simulink model "TST_TSDa_tClnt"  (R2016b)
settings: Solver=FixedStepDiscrete  StartTime=0.0  StopTime=simTime  FixedStep=sampleTime  RelTol=1e-3
values from neighbouring files (symbols this model uses):
  testCase = 1    [initTST_TSDa_tClnt_001.m]
libraries: simulink x5, UnitTest_Lib x3
settings Model: Creator=xinchangran  LastModifiedBy=xinchangran
settings DebuggingCC: SignalRangeChecking=error

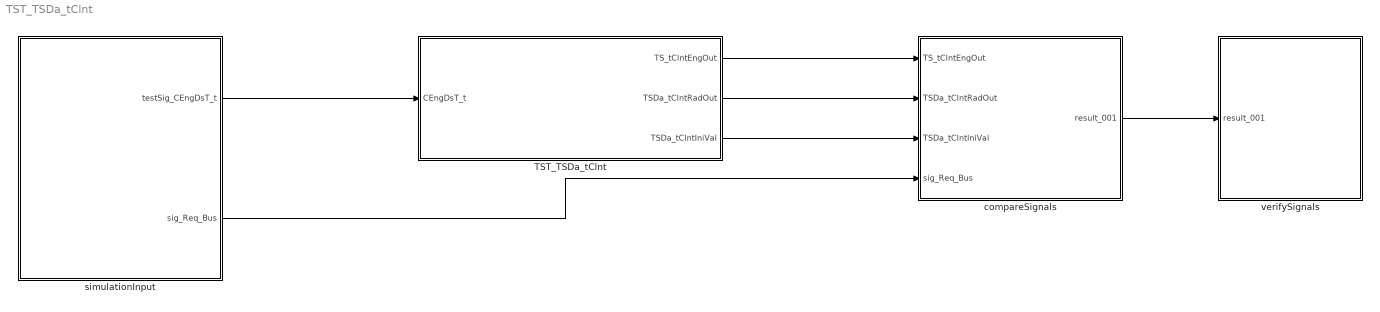
== system TST_TSDa_tClnt ==
  TST_TSDa_tClnt : Subsystem
  compareSignals : Subsystem
  simulationInput : Subsystem
  verifySignals : Subsystem
  wires:
  simulationInput/1(testSig_CEngDsT_t) -> TST_TSDa_tClnt/1(CEngDsT_t)
  TST_TSDa_tClnt/1(TS_tClntEngOut) -> compareSignals/1(TS_tClntEngOut)
  TST_TSDa_tClnt/2(TSDa_tClntRadOut) -> compareSignals/2(TSDa_tClntRadOut)
  TST_TSDa_tClnt/3(TSDa_tClntIniVal) -> compareSignals/3(TSDa_tClntIniVal)
  simulationInput/2(sig_Req_Bus) -> compareSignals/4(sig_Req_Bus)
  compareSignals/1(result_001) -> verifySignals/1(result_001)

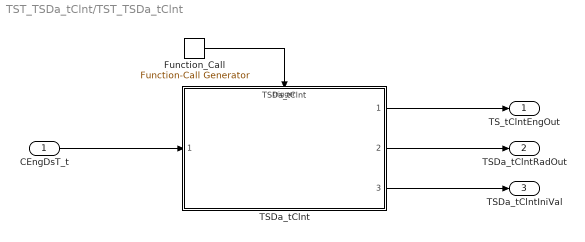
== system TST_TSDa_tClnt/TST_TSDa_tClnt ==
  CEngDsT_t : Inport
  Function_Call : simulink/Ports & Subsystems/Function-Call Generator  sample_time=sampleTime  numberOfIterations=1
  TSDa_tClnt : ModelReference  ModelNameDialog=TSDa_tClnt  SimulationMode=Normal  ModelReferenceVersion=1.10  TriggerPortName=function  TriggerPortTriggerType=function-call  TriggerPortStatesWhenEnabling=held
  TS_tClntEngOut : Outport
  TSDa_tClntRadOut : Outport  Port=2
  TSDa_tClntIniVal : Outport  Port=3
  wires:
  Function_Call/1 -> TSDa_tClnt/Trigger
  CEngDsT_t/1 -> TSDa_tClnt/1
  TSDa_tClnt/1 -> TS_tClntEngOut/1
  TSDa_tClnt/2 -> TSDa_tClntRadOut/1
  TSDa_tClnt/3 -> TSDa_tClntIniVal/1

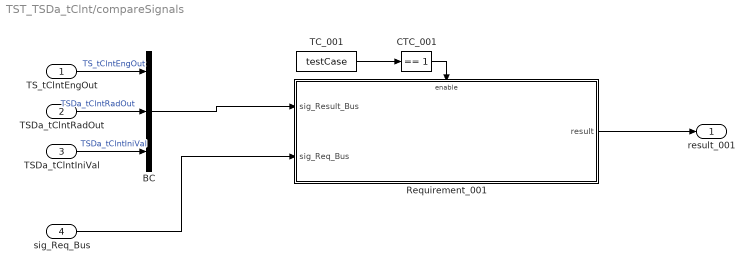
== system TST_TSDa_tClnt/compareSignals ==
  TS_tClntEngOut : Inport
  TSDa_tClntRadOut : Inport  Port=2
  TSDa_tClntIniVal : Inport  Port=3
  sig_Req_Bus : Inport  Port=4
  BC : BusCreator  Inputs=3
  CTC_001 : simulink/Logic and Bit Operations/Compare To Constant  relop===  const=1  OutDataTypeStr=boolean
  Requirement_001 : Subsystem
  TC_001 : Constant  Value=testCase
  result_001 : Outport
  wires:
  TS_tClntEngOut/1 -> BC/1  "TS_tClntEngOut"
  TSDa_tClntRadOut/1 -> BC/2  "TSDa_tClntRadOut"
  TSDa_tClntIniVal/1 -> BC/3  "TSDa_tClntIniVal"
  TC_001/1 -> CTC_001/1
  CTC_001/1 -> Requirement_001/Enable
  sig_Req_Bus/1 -> Requirement_001/2(sig_Req_Bus)
  BC/1 -> Requirement_001/1(sig_Result_Bus)
  Requirement_001/1(result) -> result_001/1

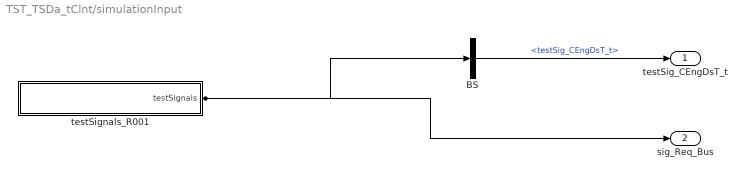
== system TST_TSDa_tClnt/simulationInput ==
  BS : BusSelector  OutputSignals=testSig_CEngDsT_t
  testSignals_R001 : Subsystem
  testSig_CEngDsT_t : Outport
  sig_Req_Bus : Outport  Port=2
  wires:
  BS/1 -> testSig_CEngDsT_t/1  "<testSig_CEngDsT_t>"
  testSignals_R001/1(testSignals) -> BS/1, sig_Req_Bus/1

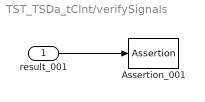
== system TST_TSDa_tClnt/verifySignals ==
  result_001 : Inport
  Assertion_001 : Assertion  Enabled=off
  wires:
  result_001/1 -> Assertion_001/1

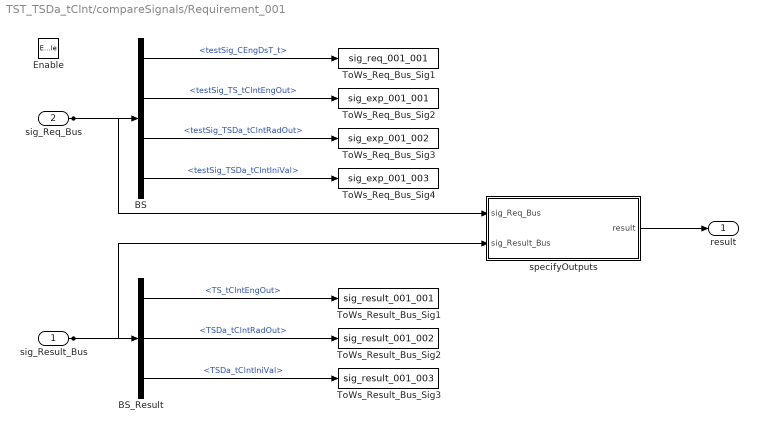
== system TST_TSDa_tClnt/compareSignals/Requirement_001 ==
  sig_Result_Bus : Inport
  sig_Req_Bus : Inport  Port=2
  Enable : EnablePort
  BS : BusSelector  OutputSignals=testSig_CEngDsT_t,testSig_TS_tClntEngOut,testSig_TSDa_tClntRadOut,testSig_TSDa_tClntIniVal
  BS_Result : BusSelector  OutputSignals=TS_tClntEngOut,TSDa_tClntRadOut,TSDa_tClntIniVal
  ToWs_Req_Bus_Sig1 : ToWorkspace  VariableName=sig_req_001_001  SaveFormat=Structure With Time
  ToWs_Req_Bus_Sig2 : ToWorkspace  VariableName=sig_exp_001_001  SaveFormat=Structure With Time
  ToWs_Req_Bus_Sig3 : ToWorkspace  VariableName=sig_exp_001_002  SaveFormat=Structure With Time
  ToWs_Req_Bus_Sig4 : ToWorkspace  VariableName=sig_exp_001_003  SaveFormat=Structure With Time
  ToWs_Result_Bus_Sig1 : ToWorkspace  VariableName=sig_result_001_001  SaveFormat=Structure With Time
  ToWs_Result_Bus_Sig2 : ToWorkspace  VariableName=sig_result_001_002  SaveFormat=Structure With Time
  ToWs_Result_Bus_Sig3 : ToWorkspace  VariableName=sig_result_001_003  SaveFormat=Structure With Time
  specifyOutputs : Subsystem
  result : Outport
  wires:
  sig_Req_Bus/1 -> BS/1, specifyOutputs/1(sig_Req_Bus)
  BS/1 -> ToWs_Req_Bus_Sig1/1  "<testSig_CEngDsT_t>"
  BS/2 -> ToWs_Req_Bus_Sig2/1  "<testSig_TS_tClntEngOut>"
  BS/3 -> ToWs_Req_Bus_Sig3/1  "<testSig_TSDa_tClntRadOut>"
  BS/4 -> ToWs_Req_Bus_Sig4/1  "<testSig_TSDa_tClntIniVal>"
  sig_Result_Bus/1 -> BS_Result/1, specifyOutputs/2(sig_Result_Bus)
  BS_Result/1 -> ToWs_Result_Bus_Sig1/1  "<TS_tClntEngOut>"
  BS_Result/2 -> ToWs_Result_Bus_Sig2/1  "<TSDa_tClntRadOut>"
  BS_Result/3 -> ToWs_Result_Bus_Sig3/1  "<TSDa_tClntIniVal>"
  specifyOutputs/1(result) -> result/1

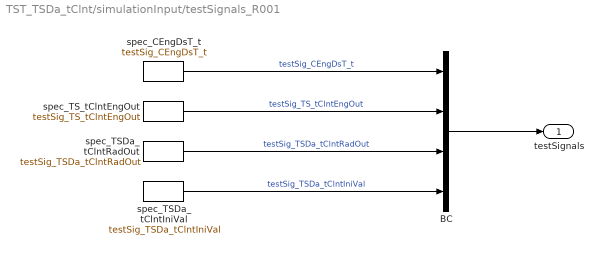
== system TST_TSDa_tClnt/simulationInput/testSignals_R001 ==
  BC : BusCreator  Inputs=4
  spec_CEngDsT_t : FromWorkspace  VariableName=testSig_CEngDsT_t  Interpolate=off  OutputAfterFinalValue=Holding final value
  spec_TSDa_tClntIniVal : FromWorkspace  VariableName=testSig_TSDa_tClntIniVal  Interpolate=off  OutputAfterFinalValue=Holding final value
  spec_TSDa_tClntRadOut : FromWorkspace  VariableName=testSig_TSDa_tClntRadOut  Interpolate=off  OutputAfterFinalValue=Holding final value
  spec_TS_tClntEngOut : FromWorkspace  VariableName=testSig_TS_tClntEngOut  Interpolate=off  OutputAfterFinalValue=Holding final value
  testSignals : Outport
  wires:
  BC/1 -> testSignals/1
  spec_CEngDsT_t/1 -> BC/1  "testSig_CEngDsT_t"
  spec_TS_tClntEngOut/1 -> BC/2  "testSig_TS_tClntEngOut"
  spec_TSDa_tClntRadOut/1 -> BC/3  "testSig_TSDa_tClntRadOut"
  spec_TSDa_tClntIniVal/1 -> BC/4  "testSig_TSDa_tClntIniVal"

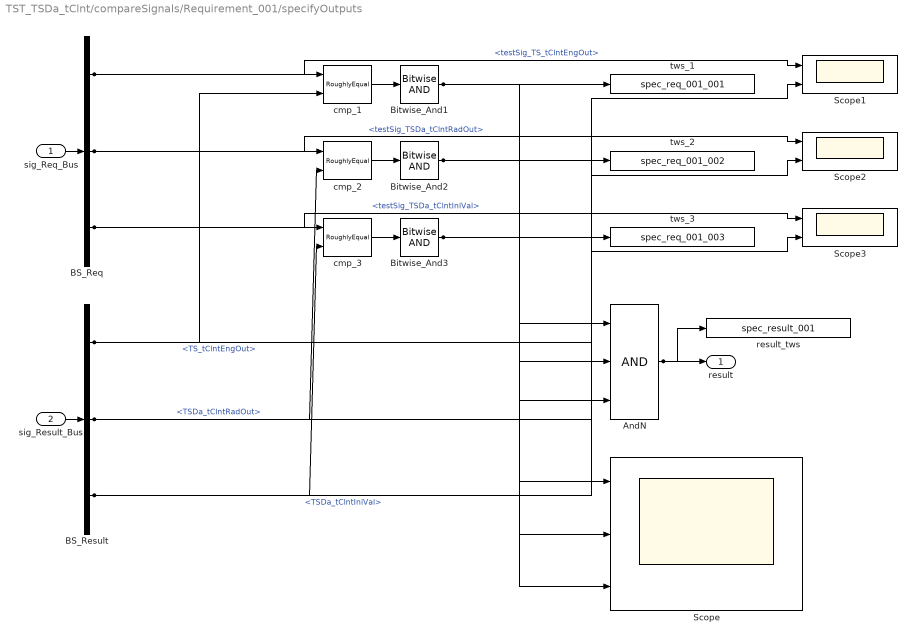
== system TST_TSDa_tClnt/compareSignals/Requirement_001/specifyOutputs ==
  sig_Req_Bus : Inport
  sig_Result_Bus : Inport  Port=2
  AndN : Logic  Inputs=3
  BS_Req : BusSelector  OutputSignals=testSig_TS_tClntEngOut,testSig_TSDa_tClntRadOut,testSig_TSDa_tClntIniVal
  BS_Result : BusSelector  OutputSignals=TS_tClntEngOut,TSDa_tClntRadOut,TSDa_tClntIniVal
  Bitwise_And1 : simulink/Logic and Bit Operations/Bitwise Operator  logicop=AND  UseBitMask=off  BitMask=bin2dec('11011001')  BitMaskRealWorld=Stored Integer
  Bitwise_And2 : simulink/Logic and Bit Operations/Bitwise Operator  logicop=AND  UseBitMask=off  BitMask=bin2dec('11011001')  BitMaskRealWorld=Stored Integer
  Bitwise_And3 : simulink/Logic and Bit Operations/Bitwise Operator  logicop=AND  UseBitMask=off  BitMask=bin2dec('11011001')  BitMaskRealWorld=Stored Integer
  Scope : Scope  NumInputPorts=3
  Scope1 : Scope  NumInputPorts=2
  Scope2 : Scope  NumInputPorts=2
  Scope3 : Scope  NumInputPorts=2
  cmp_1 : UnitTest_Lib/RoughlyEqual  slope=0.1
  cmp_2 : UnitTest_Lib/RoughlyEqual  slope=0.1
  cmp_3 : UnitTest_Lib/RoughlyEqual  slope=0.1
  result_tws : ToWorkspace  VariableName=spec_result_001
  tws_1 : ToWorkspace  VariableName=spec_req_001_001
  tws_2 : ToWorkspace  VariableName=spec_req_001_002
  tws_3 : ToWorkspace  VariableName=spec_req_001_003
  result : Outport
  wires:
  sig_Req_Bus/1 -> BS_Req/1
  sig_Result_Bus/1 -> BS_Result/1
  AndN/1 -> result/1, result_tws/1
  BS_Req/1 -> cmp_1/1, Scope1/1  "<testSig_TS_tClntEngOut>"
  BS_Result/1 -> cmp_1/2, Scope1/2  "<TS_tClntEngOut>"
  cmp_1/1 -> Bitwise_And1/1
  Bitwise_And1/1 -> tws_1/1, AndN/1, Scope/1
  BS_Req/2 -> cmp_2/1, Scope2/1  "<testSig_TSDa_tClntRadOut>"
  BS_Result/2 -> cmp_2/2, Scope2/2  "<TSDa_tClntRadOut>"
  cmp_2/1 -> Bitwise_And2/1
  Bitwise_And2/1 -> tws_2/1, AndN/2, Scope/2
  BS_Req/3 -> cmp_3/1, Scope3/1  "<testSig_TSDa_tClntIniVal>"
  BS_Result/3 -> cmp_3/2, Scope3/2  "<TSDa_tClntIniVal>"
  cmp_3/1 -> Bitwise_And3/1
  Bitwise_And3/1 -> tws_3/1, AndN/3, Scope/3
